simulink model "Intro2Robotics9"  (R2014a)
settings: Solver=ode45  StartTime=0.0  StopTime=5  RelTol=1e-3
libraries: simulink x3
settings Model: Creator=HUANGJing  LastModifiedBy=HUANGJing

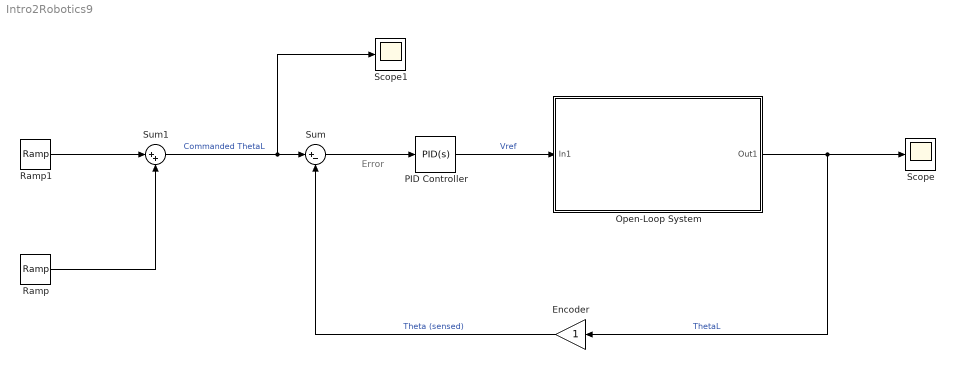
== system Intro2Robotics9 ==
  note: Error
  Encoder : Gain
  Open-Loop System : Subsystem
  PID Controller : simulink/Continuous/PID Controller  Controller=PID  TimeDomain=Continuous-time  SampleTime=1  IntegratorMethod=Forward Euler  FilterMethod=Forward Euler  Form=Parallel  P=0.926572977871014  I=0.313415482239011  D=0.217125556055133  N=9.90736610664397  InitialConditionSource=internal  InitialConditionForIntegrator=0  InitialConditionForFilter=0  ExternalReset=none  LimitOutput=off  UpperSaturationLimit=inf  LowerSaturationLimit=-inf  LinearizeAsGain=on  AntiWindupMode=none  Kb=1  TrackingMode=off  Kt=1  PParamMin=[]  PParamMax=[]  IParamMin=[]  IParamMax=[]  DParamMin=[]  DParamMax=[]  NParamMin=[]  NParamMax=[]  KbParamMin=[]  KbParamMax=[]  KtParamMin=[]  KtParamMax=[]  POutMin=[]  POutMax=[]  IOutMin=[]  IOutMax=[]  DOutMin=[]  DOutMax=[]  NOutMin=[]  NOutMax=[]  KbOutMin=[]  KbOutMax=[]  KtOutMin=[]  KtOutMax=[]  IntegratorOutMin=[]  IntegratorOutMax=[]  FilterOutMin=[]  FilterOutMax=[]  SumOutMin=[]  SumOutMax=[]  SumI1OutMin=[]  SumI1OutMax=[]  SumI2OutMin=[]  SumI2OutMax=[]  SumI3OutMin=[]  SumI3OutMax=[]  SumDOutMin=[]  SumDOutMax=[]  SaturationOutMin=[]  SaturationOutMax=[]  IntegratorContinuousStateAttributes=''  IntegratorStateMustResolveToSignalObject=off  IntegratorRTWStateStorageClass=Auto  FilterContinuousStateAttributes=''  FilterStateMustResolveToSignalObject=off  FilterRTWStateStorageClass=Auto
  Ramp : simulink/Sources/Ramp  slope=40  start=0  X0=0
  Ramp1 : simulink/Sources/Ramp  slope=-40  start=1.5  X0=0
  Scope : Scope
  Scope1 : Scope
  Sum : Sum  Inputs=|+-
  Sum1 : Sum  Inputs=|++
  wires:
  PID Controller/1 -> Open-Loop System/1(In1)  "Vref"
  Open-Loop System/1(Out1) -> Encoder/1, Scope/1  "ThetaL"
  Sum/1 -> PID Controller/1
  Encoder/1 -> Sum/2  "Theta (sensed)"
  Sum1/1 -> Scope1/1, Sum/1  "Commanded ThetaL"
  Ramp/1 -> Sum1/2
  Ramp1/1 -> Sum1/1

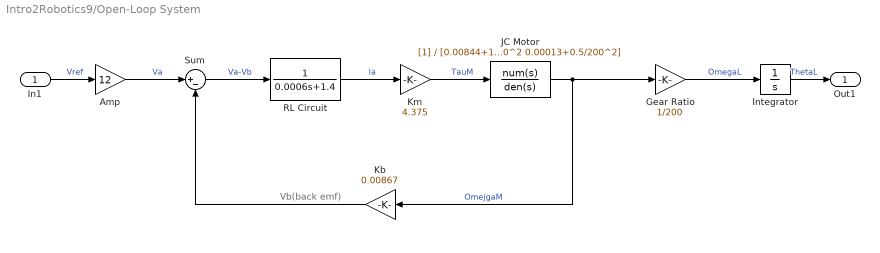
== system Intro2Robotics9/Open-Loop System ==
  note: Vb(back emf)
  In1 : Inport
  Amp : Gain  Gain=12
  Gear Ratio : Gain  Gain=1/200
  Integrator : Integrator
  JC Motor : TransferFcn  Denominator=[0.00844+1/200^2 0.00013+0.5/200^2]
  Kb : Gain  Gain=0.00867
  Km : Gain  Gain=4.375
  RL Circuit : TransferFcn  Denominator=[0.0006 1.4]
  Sum : Sum  Inputs=|+-
  Out1 : Outport
  wires:
  Kb/1 -> Sum/2
  Sum/1 -> RL Circuit/1  "Va-Vb"
  Gear Ratio/1 -> Integrator/1  "OmegaL"
  RL Circuit/1 -> Km/1  "la"
  JC Motor/1 -> Kb/1, Gear Ratio/1  "OmejgaM"
  Km/1 -> JC Motor/1  "TauM"
  Amp/1 -> Sum/1  "Va"
  Integrator/1 -> Out1/1  "ThetaL"
  In1/1 -> Amp/1  "Vref"
